simulink model "sideslip_loop"  (R2016b)
settings: Solver=VariableStepAuto  StartTime=0.0  StopTime=10.0  RelTol=1e-3
undefined symbols (not defined in the file): a_beta1, a_beta2, k_i_beta, k_p_beta
settings Model: Creator=geun2  LastModifiedBy=geun2

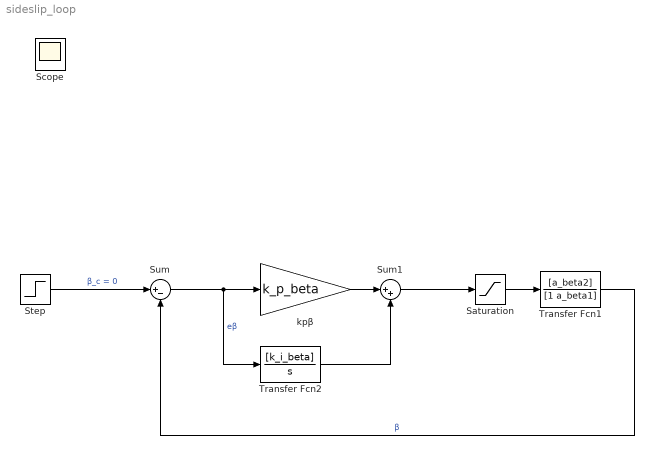
== system sideslip_loop ==
  Saturation : Saturate  UpperLimit=20*pi/180  LowerLimit=-20*pi/180
  Step : Step  After=3*pi/180  SampleTime=0
  Sum : Sum  Inputs=|+-
  Sum1 : Sum  Inputs=|++
  Transfer Fcn1 : TransferFcn  Numerator=[a_beta2]  Denominator=[1 a_beta1]
  Transfer Fcn2 : TransferFcn  Numerator=[k_i_beta]  Denominator=[1 0]
  kpβ : Gain  Gain=k_p_beta
  Scope : Scope
  wires:
  Sum/1 -> Transfer Fcn2/1, kpβ/1  "eβ"
  Transfer Fcn1/1 -> Sum/2  "β"
  Step/1 -> Sum/1  "β_c = 0"
  kpβ/1 -> Sum1/1
  Transfer Fcn2/1 -> Sum1/2
  Sum1/1 -> Saturation/1
  Saturation/1 -> Transfer Fcn1/1
